simulink model "SumaDosVariables"  (R2021b)
settings: Solver=FixedStepAuto  StartTime=0.0  StopTime=1  FixedStep=0.5  RelTol=1e-3
undefined symbols (not defined in the file or in its folder): k
settings Model: Creator=mluser  LastModifiedBy=mluser

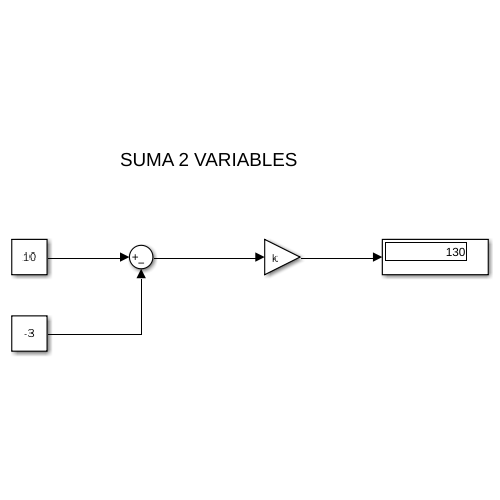
[thumbnail: Simulink's stored preview of the top-level diagram]
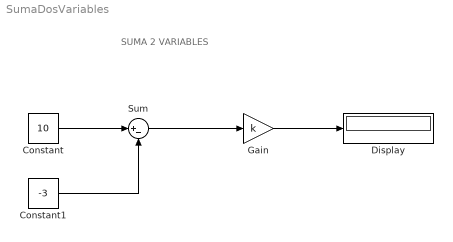
== system SumaDosVariables ==
  note: SUMA 2 VARIABLES
  Constant : Constant  Value=10
  Constant1 : Constant  Value=-3
  Display : Display
  Gain : Gain  Gain=k
  Sum : Sum  Inputs=|+-
  wires:
  Constant/1 -> Sum/1
  Constant1/1 -> Sum/2
  Sum/1 -> Gain/1
  Gain/1 -> Display/1
